simulink model "Task_6_2"  (R2015a)
settings: Solver=ode45  StartTime=0.0  StopTime=10.0  RelTol=1e-3
undefined symbols (not defined in the file): x
settings Model: Creator=acer  LastModifiedBy=acer

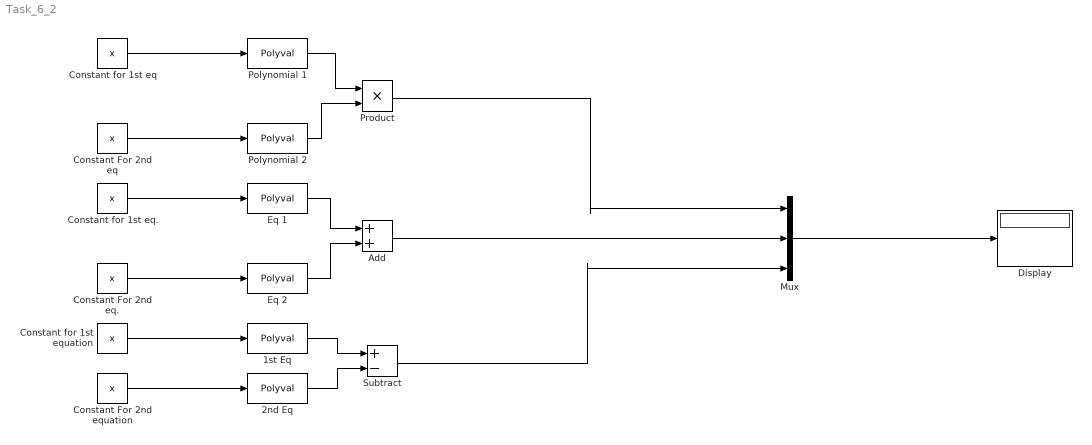
== system Task_6_2 ==
  1st Eq : Polyval  Coefs=[ 1 0 4 2 7 1 ]
  2nd Eq : Polyval  Coefs=[ 4 2 0 0 0]
  Add : Sum
  Constant For 2nd eq : Constant  Value=x
  Constant For 2nd eq. : Constant  Value=x
  Constant For 2nd equation : Constant  Value=x
  Constant for 1st eq : Constant  Value=x
  Constant for 1st eq. : Constant  Value=x
  Constant for 1st equation : Constant  Value=x
  Display : Display
  Eq 1 : Polyval  Coefs=[ 1 0 4 2 7 1 ]
  Eq 2 : Polyval  Coefs=[ 4 2 0 0 0]
  Mux : Mux  Inputs=3
  Polynomial 1 : Polyval  Coefs=[ 1 0 4 2 7 1 ]
  Polynomial 2 : Polyval  Coefs=[ 4 2 0 0 0]
  Product : Product
  Subtract : Sum  Inputs=+-
  wires:
  Constant for 1st eq/1 -> Polynomial 1/1
  Constant For 2nd eq/1 -> Polynomial 2/1
  Constant for 1st eq./1 -> Eq 1/1
  Constant For 2nd eq./1 -> Eq 2/1
  Constant for 1st equation/1 -> 1st Eq/1
  Constant For 2nd equation/1 -> 2nd Eq/1
  Eq 1/1 -> Add/1
  Eq 2/1 -> Add/2
  Polynomial 1/1 -> Product/1
  Polynomial 2/1 -> Product/2
  1st Eq/1 -> Subtract/1
  2nd Eq/1 -> Subtract/2
  Product/1 -> Mux/1
  Add/1 -> Mux/2
  Subtract/1 -> Mux/3
  Mux/1 -> Display/1
